simulink model "firstorderdcmotor"  (R2025b)
settings: Solver=VariableStepAuto  StartTime=0.0  StopTime=10.0  RelTol=1e-3
settings Model: Creator=daryl  LastModifiedBy=daryl

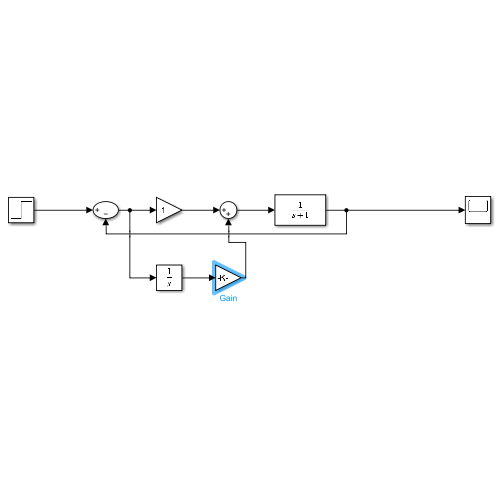
[thumbnail: Simulink's stored preview of the top-level diagram]
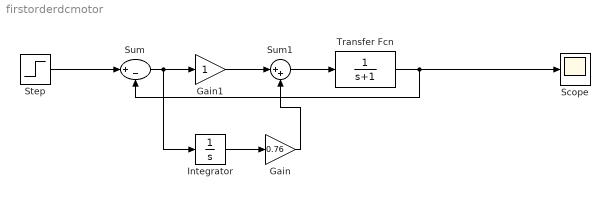
== system firstorderdcmotor ==
  Gain : Gain  Gain=0.76
  Gain1 : Gain
  Integrator : Integrator
  Scope : Scope
      settings: ActiveDisplayYMinimum=-247.31952232680419  ActiveDisplayYMaximum=1476.0036568082251
  Step : Step  After=1000  SampleTime=0
  Sum : Sum  Inputs=|+-
  Sum1 : Sum  Inputs=|++
  Transfer Fcn : TransferFcn  Denominator=[1 1]
  wires:
  Step/1 -> Sum/1
  Sum/1 -> Gain1/1, Integrator/1
  Sum1/1 -> Transfer Fcn/1
  Integrator/1 -> Gain/1
  Gain/1 -> Sum1/2
  Transfer Fcn/1 -> Scope/1, Sum/2
  Gain1/1 -> Sum1/1
